simulink model "Ather_Powertrain"  (R2020a)
settings: Solver=FixedStepAuto  StartTime=0.0  StopTime=993  FixedStep=0.5  RelTol=1e-3
values from neighbouring files (symbols this model uses):
  A = 0.875    [imports.m]
  B_Voltage = 51.1    [imports.m]
  Ccap = 2.7    [imports.m]
  Cd = 0.22    [imports.m]
  Crf = 0.015    [imports.m]
  Cv = 3.6    [imports.m]
  Distance = 14.03    [imports.m]
  GR = 7.8    [imports.m]
  GVM = M+Md    (= 191)    [imports.m]
  GVW = GVM * g    (= 1873.71)    [imports.m]
  ISOC = 1    [imports.m]
  MController_Eff = 85    [imports.m]
  Motor_Eff = 90    [imports.m]
  Neff = 0.85    [imports.m]
  rho = 1.225    [imports.m]
  Rw = 0.1524    [imports.m]
settings Model: Creator=HP  LastModifiedBy=HP

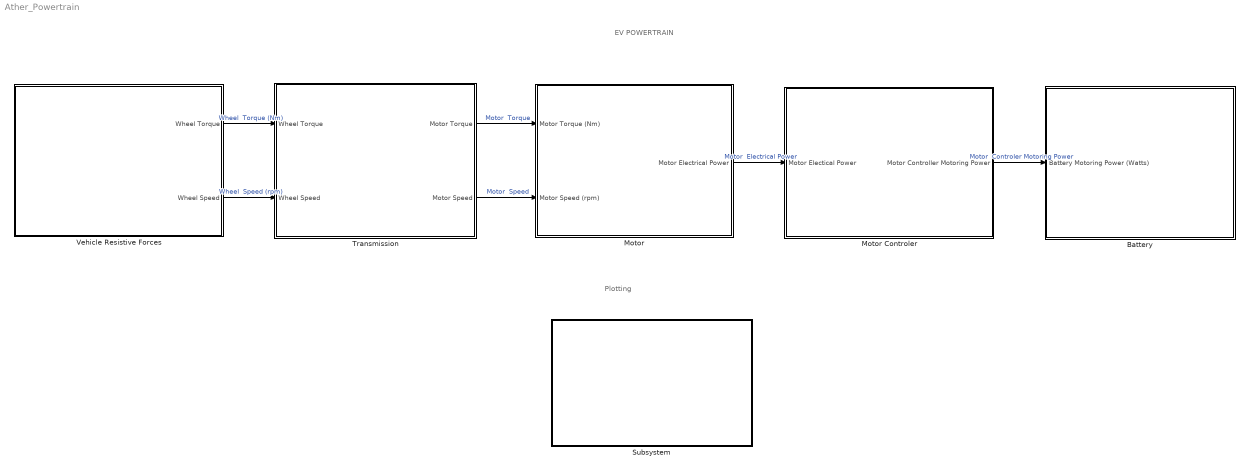
== system Ather_Powertrain ==
  note: EV POWERTRAIN
  note: Plotting
  Battery : Subsystem
      mask Display: image('C:\Users\HP\Pictures\Capture4.PNG'); % Use "Edit Image" on toolstrip to change.
  Motor : Subsystem
      mask Display: image('C:\Users\HP\Pictures\Capture3.PNG'); % Use "Edit Image" on toolstrip to change.
  Motor Controler : Subsystem
      mask Display: image('C:\Users\HP\Downloads\c.jpg'); % Use "Edit Image" on toolstrip to change.
  Subsystem : Subsystem
      mask Display: image('C:\Users\HP\Downloads\g.png'); % Use "Edit Image" on toolstrip to change.
  Transmission : Subsystem
      mask Display: image('C:\Users\HP\Pictures\Capture2.PNG'); % Use "Edit Image" on toolstrip to change.
  Vehicle Resistive Forces : Subsystem
      mask Display: image('C:\Users\HP\Pictures\Capture.PNG'); % Use "Edit Image" on toolstrip to change.
  wires:
  Vehicle Resistive Forces/1(Wheel Torque) -> Transmission/1(Wheel Torque)  "Wheel  Torque (Nm)"
  Vehicle Resistive Forces/2(Wheel Speed) -> Transmission/2(Wheel Speed)  "Wheel  Speed (rpm)"
  Transmission/1(Motor Torque) -> Motor/1(Motor Torque (Nm))  "Motor  Torque"
  Transmission/2(Motor Speed) -> Motor/2(Motor Speed (rpm))  "Motor  Speed"
  Motor/1(Motor Electrical Power) -> Motor Controler/1(Motor Electical Power)  "Motor  Electrical Power"
  Motor Controler/1(Motor Controller Motoring Power) -> Battery/1(Battery Motoring Power (Watts))  "Motor  Controler Motoring Power"

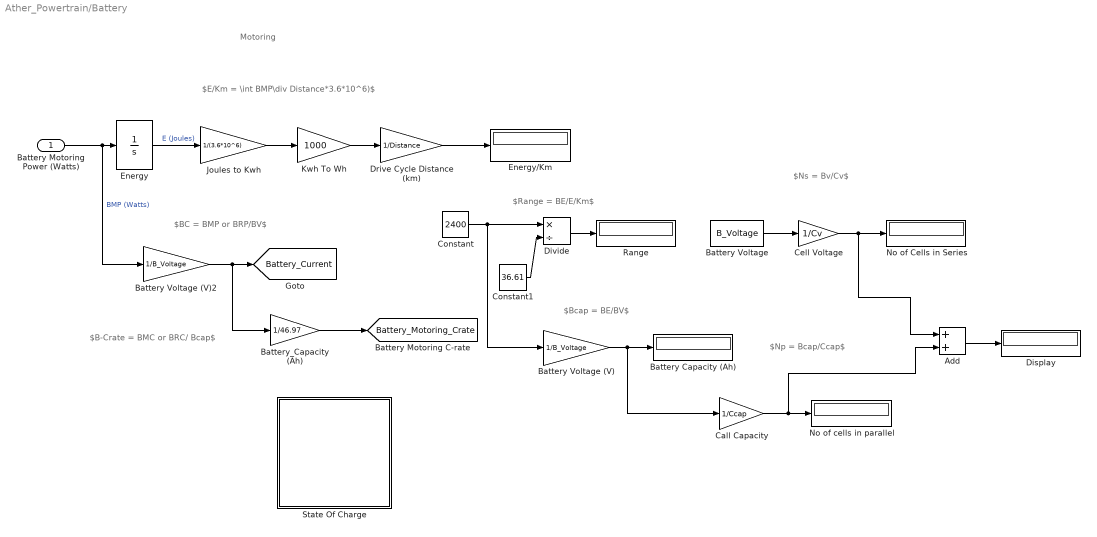
== system Ather_Powertrain/Battery ==
  note: $Np = Bcap/Ccap$
  note: $Ns = Bv/Cv$
  note: Motoring
  note: $B-Crate = BMC or BRC/ Bcap$
  note: $BC = BMP or BRP/BV$
  note: $Bcap = BE/BV$
  note: $Range = BE/E/Km$
  note: $E/Km = \int BMP\div Distance*3.6*10^6)$
  Battery Motoring Power (Watts) : Inport
  Add : Sum
  Battery Capacity (Ah) : Display
  Battery Voltage : Constant  Value=B_Voltage
  Battery Voltage (V) : Gain  Gain=1/B_Voltage
  Battery Voltage (V)2 : Gain  Gain=1/B_Voltage
  Battery_Capacity (Ah) : Gain  Gain=1/46.97
  Call Capacity : Gain  Gain=1/Ccap
  Cell Voltage : Gain  Gain=1/Cv
  Constant : Constant  Value=2400
  Constant1 : Constant  Value=36.61
  Display : Display
  Divide : Product  Inputs=*/
  Drive Cycle Distance (km) : Gain  Gain=1/Distance
  Energy : Integrator
  Energy/Km : Display
  Joules to Kwh : Gain  Gain=1/(3.6*10^6)
  Kwh To Wh : Gain  Gain=1000
  No of Cells in Series : Display
  No of cells in parallel : Display
  Range : Display
  State Of Charge : Subsystem
  tag scope: Battery_Current=global, Battery_Motoring_Crate=global
  wires:
  Battery Motoring Power (Watts)/1 -> Battery Voltage (V)2/1, Energy/1  "BMP (Watts)"
  Energy/1 -> Joules to Kwh/1  "E (Joules)"
  Joules to Kwh/1 -> Kwh To Wh/1
  Kwh To Wh/1 -> Drive Cycle Distance (km)/1
  Drive Cycle Distance (km)/1 -> Energy/Km/1
  Battery Voltage (V)/1 -> Call Capacity/1, Battery Capacity (Ah)/1
  Battery Voltage (V)2/1 -> Battery_Capacity (Ah)/1, [Battery_Current]
  Battery_Capacity (Ah)/1 -> [Battery_Motoring_Crate]
  Cell Voltage/1 -> Add/1, No of Cells in Series/1
  Battery Voltage/1 -> Cell Voltage/1
  Call Capacity/1 -> Add/2, No of cells in parallel/1
  Constant1/1 -> Divide/2
  Constant/1 -> Battery Voltage (V)/1, Divide/1
  Divide/1 -> Range/1
  Add/1 -> Display/1

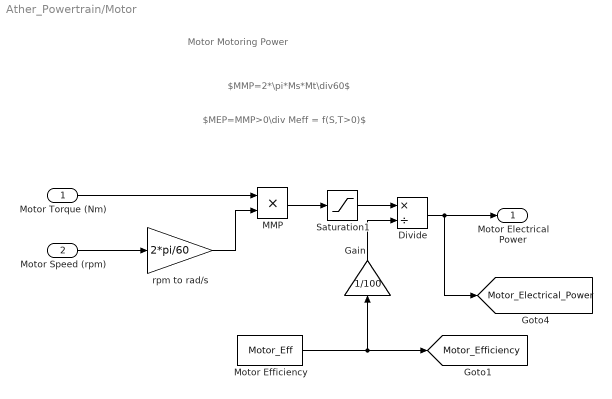
== system Ather_Powertrain/Motor ==
  note: Motor Motoring Power
  note: $MEP=MMP>0\div Meff = f(S,T>0)$
  note: $MMP=2*\pi*Ms*Mt\div60$
  Motor Torque (Nm) : Inport
  Motor Speed (rpm) : Inport  Port=2
  Divide : Product  Inputs=*/
  Gain : Gain  Gain=1/100
  MMP : Product
  Motor Efficiency : Constant  Value=Motor_Eff
  Saturation1 : Saturate  UpperLimit=Inf  LowerLimit=0
  rpm to rad/s : Gain  Gain=2*pi/60
  Motor Electrical Power : Outport
  tag scope: Motor_Efficiency=global, Motor_Electrical_Power=global
  wires:
  Motor Torque (Nm)/1 -> MMP/1
  rpm to rad/s/1 -> MMP/2
  Motor Speed (rpm)/1 -> rpm to rad/s/1
  Motor Efficiency/1 -> [Motor_Efficiency], Gain/1
  Gain/1 -> Divide/2
  MMP/1 -> Saturation1/1
  Divide/1 -> [Motor_Electrical_Power], Motor Electrical Power/1
  Saturation1/1 -> Divide/1

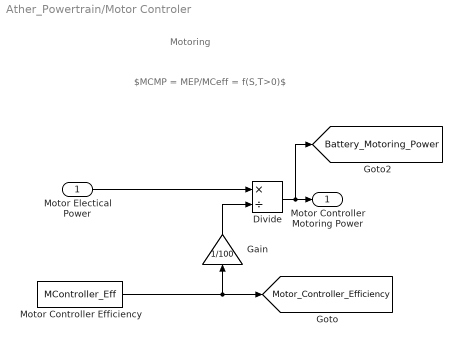
== system Ather_Powertrain/Motor Controler ==
  note: Motoring
  note: $MCMP = MEP/MCeff = f(S,T>0)$
  Motor Electical Power : Inport
  Divide : Product  Inputs=*/
  Gain : Gain  Gain=1/100
  Motor Controller Efficiency : Constant  Value=MController_Eff
  Motor Controller Motoring Power : Outport
  tag scope: Battery_Motoring_Power=global, Motor_Controller_Efficiency=global
  wires:
  Divide/1 -> [Battery_Motoring_Power], Motor Controller Motoring Power/1
  Motor Controller Efficiency/1 -> Gain/1, [Motor_Controller_Efficiency]
  Gain/1 -> Divide/2
  Motor Electical Power/1 -> Divide/1

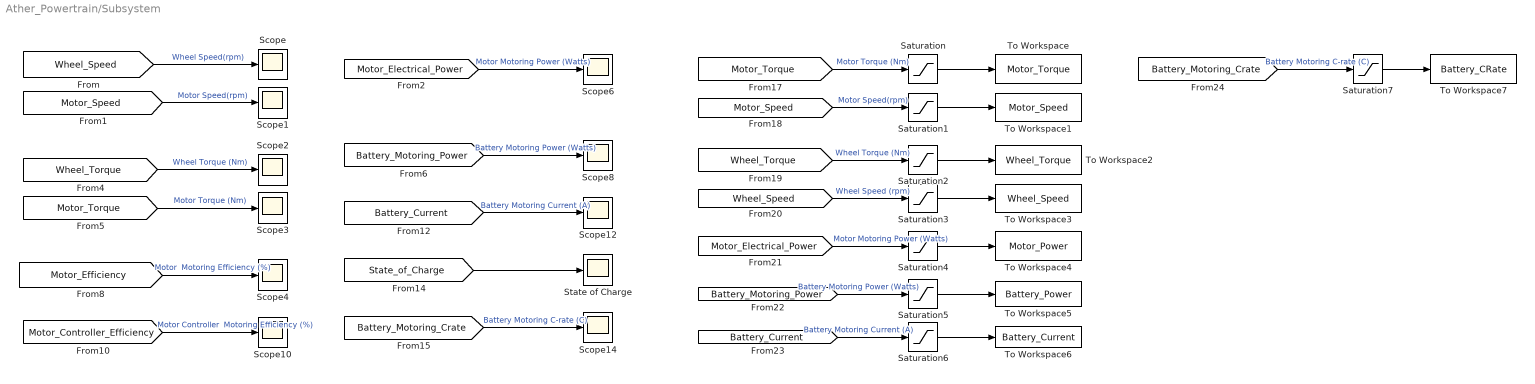
== system Ather_Powertrain/Subsystem ==
  Saturation{,1..7} (8 alike) : Saturate  UpperLimit=inf  LowerLimit=0
  Scope{,1..4,6,8,10,12,14} (10 alike) : Scope
  State of Charge : Scope
  To Workspace : ToWorkspace  VariableName=Motor_Torque  SaveFormat=Timeseries  SampleTime=-1
  To Workspace1 : ToWorkspace  VariableName=Motor_Speed  SaveFormat=Timeseries  SampleTime=-1
  To Workspace2 : ToWorkspace  VariableName=Wheel_Torque  SaveFormat=Timeseries  SampleTime=-1
  To Workspace3 : ToWorkspace  VariableName=Wheel_Speed  SaveFormat=Timeseries  SampleTime=-1
  To Workspace4 : ToWorkspace  VariableName=Motor_Power  SaveFormat=Timeseries  SampleTime=-1
  To Workspace5 : ToWorkspace  VariableName=Battery_Power  SaveFormat=Timeseries  SampleTime=-1
  To Workspace6 : ToWorkspace  VariableName=Battery_Current  SaveFormat=Timeseries  SampleTime=-1
  To Workspace7 : ToWorkspace  VariableName=Battery_CRate  SaveFormat=Timeseries  SampleTime=-1
  wires:
  Saturation/1 -> To Workspace/1
  [Wheel_Speed] -> Saturation3/1  "Wheel Speed (rpm)"
  [Motor_Electrical_Power] -> Scope6/1  "Motor Motoring Power (Watts)"
  [Wheel_Torque] -> Scope2/1  "Wheel Torque (Nm)"
  Saturation6/1 -> To Workspace6/1
  [Motor_Controller_Efficiency] -> Scope10/1  "Motor Controller  Motoring Efficiency (%)"
  Saturation4/1 -> To Workspace4/1
  [Motor_Torque] -> Scope3/1  "Motor Torque (Nm)"
  [Battery_Motoring_Power] -> Scope8/1  "Battery Motoring Power (Watts)"
  [Battery_Motoring_Crate] -> Scope14/1  "Battery Motoring C-rate (C)"
  [Motor_Speed] -> Saturation1/1  "Motor Speed(rpm)"
  Saturation1/1 -> To Workspace1/1
  [State_of_Charge] -> State of Charge/1
  Saturation5/1 -> To Workspace5/1
  [Motor_Speed] -> Scope1/1  "Motor Speed(rpm)"
  [Wheel_Speed] -> Scope/1  "Wheel Speed(rpm)"
  [Battery_Current] -> Saturation6/1  "Battery Motoring Current (A)"
  [Motor_Efficiency] -> Scope4/1  "Motor  Motoring Efficiency (%)"
  [Battery_Current] -> Scope12/1  "Battery Motoring Current (A)"
  [Motor_Electrical_Power] -> Saturation4/1  "Motor Motoring Power (Watts)"
  Saturation2/1 -> To Workspace2/1
  Saturation3/1 -> To Workspace3/1
  [Motor_Torque] -> Saturation/1  "Motor Torque (Nm)"
  [Battery_Motoring_Crate] -> Saturation7/1  "Battery Motoring C-rate (C)"
  [Wheel_Torque] -> Saturation2/1  "Wheel Torque (Nm)"
  Saturation7/1 -> To Workspace7/1
  [Battery_Motoring_Power] -> Saturation5/1  "Battery Motoring Power (Watts)"

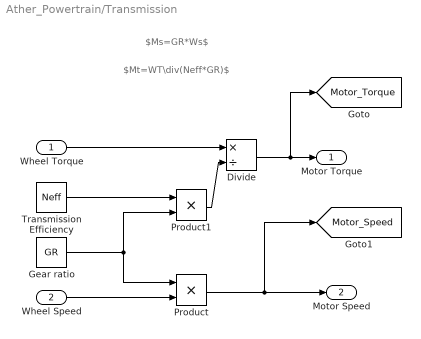
== system Ather_Powertrain/Transmission ==
  note: $Mt=WT\div(Neff*GR)$
  note: $Ms=GR*Ws$
  Wheel Torque : Inport
  Wheel Speed : Inport  Port=2
  Divide : Product  Inputs=*/
  Gear ratio : Constant  Value=GR
  Product : Product
  Product1 : Product
  Transmission Efficiency : Constant  Value=Neff
  Motor Torque : Outport
  Motor Speed : Outport  Port=2
  tag scope: Motor_Speed=global, Motor_Torque=global
  wires:
  Wheel Speed/1 -> Product/2
  Gear ratio/1 -> Product1/2, Product/1
  Product/1 -> [Motor_Speed], Motor Speed/1
  Transmission Efficiency/1 -> Product1/1
  Product1/1 -> Divide/2
  Wheel Torque/1 -> Divide/1
  Divide/1 -> [Motor_Torque], Motor Torque/1

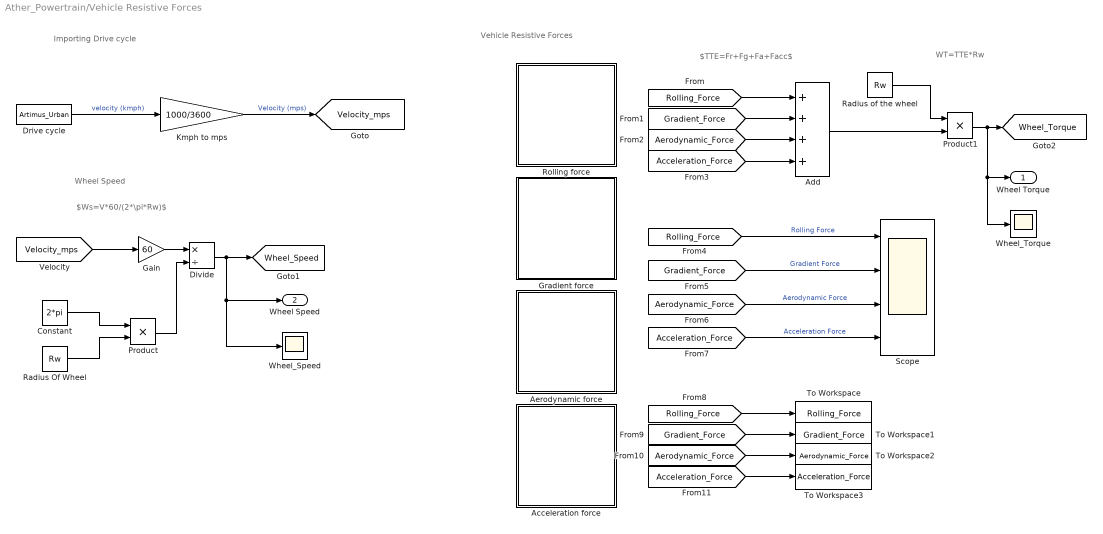
== system Ather_Powertrain/Vehicle Resistive Forces ==
  note: WT=TTE*Rw
  note: $TTE=Fr+Fg+Fa+Facc$
  note: Vehicle Resistive Forces
  note: $Ws=V*60/(2*\pi*Rw)$
  note: Wheel Speed
  note: Importing Drive cycle
  Acceleration force : Subsystem
  Add : Sum  Inputs=++++
  Aerodynamic force : Subsystem
  Constant : Constant  Value=2*pi
  Divide : Product  Inputs=*/
  Drive cycle : FromWorkspace  VariableName=Artimus_Urban
  Gain : Gain  Gain=60
  Gradient force : Subsystem
  Kmph to mps : Gain  Gain=1000/3600
  Product : Product
  Product1 : Product
  Radius Of Wheel : Constant  Value=Rw
  Radius of the wheel : Constant  Value=Rw
  Rolling force : Subsystem
  Scope : Scope  NumInputPorts=4
  To Workspace : ToWorkspace  VariableName=Rolling_Force  SaveFormat=Timeseries  SampleTime=-1
  To Workspace1 : ToWorkspace  VariableName=Gradient_Force  SaveFormat=Timeseries  SampleTime=-1
  To Workspace2 : ToWorkspace  VariableName=Aerodynamic_Force  SaveFormat=Timeseries  SampleTime=-1
  To Workspace3 : ToWorkspace  VariableName=Acceleration_Force  SaveFormat=Timeseries  SampleTime=-1
  Wheel_Speed : Scope
  Wheel_Torque : Scope
  Wheel Torque : Outport
  Wheel Speed : Outport  Port=2
  tag scope: Velocity_mps=global, Wheel_Speed=global, Wheel_Torque=global
  wires:
  Drive cycle/1 -> Kmph to mps/1  "velocity (kmph)"
  Kmph to mps/1 -> [Velocity_mps]  "Velocity (mps)"
  [Velocity_mps] -> Gain/1
  Constant/1 -> Product/1
  Radius Of Wheel/1 -> Product/2
  Gain/1 -> Divide/1
  Product/1 -> Divide/2
  Divide/1 -> Wheel_Speed/1, Wheel Speed/1, [Wheel_Speed]
  [Rolling_Force] -> Add/1
  [Gradient_Force] -> Add/2
  [Aerodynamic_Force] -> Add/3
  [Acceleration_Force] -> Add/4
  Add/1 -> Product1/2
  Radius of the wheel/1 -> Product1/1
  Product1/1 -> Wheel_Torque/1, Wheel Torque/1, [Wheel_Torque]
  [Gradient_Force] -> Scope/2  "Gradient Force"
  [Rolling_Force] -> Scope/1  "Rolling Force"
  [Aerodynamic_Force] -> Scope/3  "Aerodynamic Force"
  [Acceleration_Force] -> Scope/4  "Acceleration Force"
  [Rolling_Force] -> To Workspace/1
  [Gradient_Force] -> To Workspace1/1
  [Aerodynamic_Force] -> To Workspace2/1
  [Acceleration_Force] -> To Workspace3/1

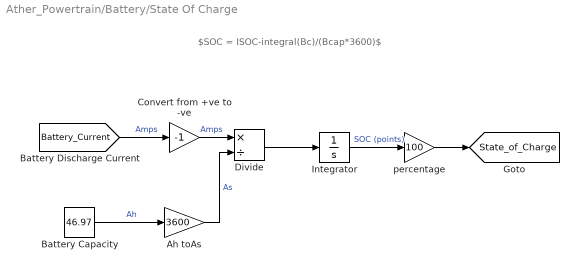
== system Ather_Powertrain/Battery/State Of Charge ==
  note: $SOC = ISOC-integral(Bc)/(Bcap*3600)$
  Ah toAs : Gain  Gain=3600
  Battery Capacity : Constant  Value=46.97
  Convert from +ve to -ve : Gain  Gain=-1
  Divide : Product  Inputs=*/
  Integrator : Integrator  InitialCondition=ISOC
  percentage : Gain  Gain=100
  tag scope: State_of_Charge=global
  wires:
  percentage/1 -> [State_of_Charge]
  [Battery_Current] -> Convert from +ve to -ve/1  "Amps"
  Battery Capacity/1 -> Ah toAs/1  "Ah"
  Ah toAs/1 -> Divide/2  "As"
  Divide/1 -> Integrator/1
  Integrator/1 -> percentage/1  "SOC (points)"
  Convert from +ve to -ve/1 -> Divide/1  "Amps"

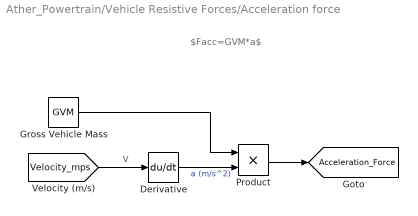
== system Ather_Powertrain/Vehicle Resistive Forces/Acceleration force ==
  note: $Facc=GVM*a$
  Derivative : Derivative
  Gross Vehicle Mass : Constant  Value=GVM
  Product : Product
  tag scope: Acceleration_Force=global
  wires:
  [Velocity_mps] -> Derivative/1  "V"
  Gross Vehicle Mass/1 -> Product/1
  Derivative/1 -> Product/2  "a (m/s^2)"
  Product/1 -> [Acceleration_Force]

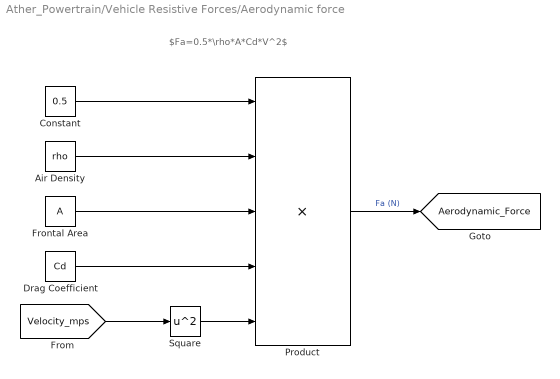
== system Ather_Powertrain/Vehicle Resistive Forces/Aerodynamic force ==
  note: $Fa=0.5*\rho*A*Cd*V^2$
  Air Density : Constant  Value=rho
  Constant : Constant  Value=0.5
  Drag Coefficient : Constant  Value=Cd
  Frontal Area : Constant  Value=A
  Product : Product  Inputs=5
  Square : Math  Operator=square  SaturateOnIntegerOverflow=on
  tag scope: Aerodynamic_Force=global
  wires:
  [Velocity_mps] -> Square/1
  Constant/1 -> Product/1
  Air Density/1 -> Product/2
  Frontal Area/1 -> Product/3
  Drag Coefficient/1 -> Product/4
  Square/1 -> Product/5
  Product/1 -> [Aerodynamic_Force]  "Fa (N)"

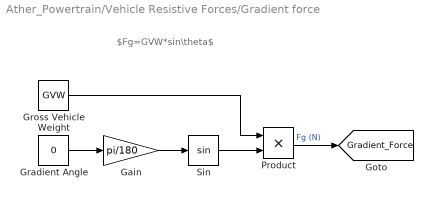
== system Ather_Powertrain/Vehicle Resistive Forces/Gradient force ==
  note: $Fg=GVW*sin\theta$
  Gain : Gain  Gain=pi/180
  Gradient Angle : Constant  Value=0
  Gross Vehicle Weight : Constant  Value=GVW
  Product : Product
  Sin : Trigonometry
  tag scope: Gradient_Force=global
  wires:
  Gradient Angle/1 -> Gain/1
  Gain/1 -> Sin/1
  Gross Vehicle Weight/1 -> Product/1
  Sin/1 -> Product/2
  Product/1 -> [Gradient_Force]  "Fg (N)"

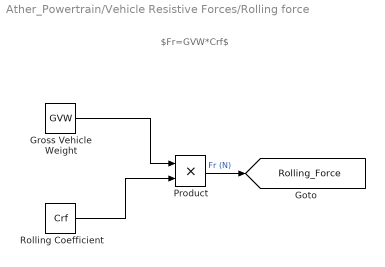
== system Ather_Powertrain/Vehicle Resistive Forces/Rolling force ==
  note: $Fr=GVW*Crf$
  Gross Vehicle Weight : Constant  Value=GVW
  Product : Product
  Rolling Coefficient : Constant  Value=Crf
  tag scope: Rolling_Force=global
  wires:
  Gross Vehicle Weight/1 -> Product/1
  Rolling Coefficient/1 -> Product/2
  Product/1 -> [Rolling_Force]  "Fr (N)"
